simulink model "motor_ctrl_reminder"  (R2020b)
settings: Solver=VariableStepAuto  StartTime=0.0  StopTime=1  RelTol=1e-3
InitFcn:
  | Rs=0.43;
  | %Ls=31.691*1e-3;
  | Lls=0.002
  | %Rr=91.9*1e-3;
  | Rr=0.816;
  | %Lr=31.093*1e-3;
  | Llr=0.002
  | %Lm=29.897*1e-3;
  | Lm=0.6931;
  | 
  | Ls = 1.5*Lm+Lls
  | Lr = 1.5*Lm+Llr
  | 
  | Tr = Lr/Rr;
  | sigma = (Ls*Lr-Lm*Lm)/Ls/Lr;
  | 
  | J=0.085;
  | np=2;
  | 
  | Ts=1e-5;
model workspace (MAT data in the model file):
  Tsys = 2e-06
  sample_time = 1e-06
libraries: powerlib x7, simulink x2
settings Model: OrderedModelArguments=off  Creator=messer  LastModifiedBy=messer

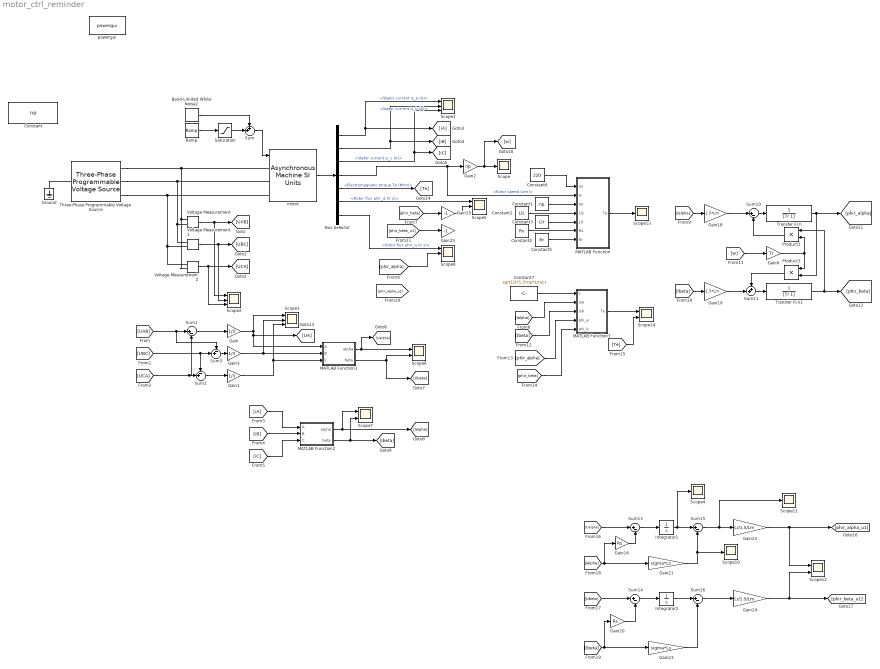
== system motor_ctrl_reminder ==
  Band-Limited White Noise2 : simulink/Sources/Band-Limited White Noise  Cov=[0.0001]  Ts=1e-4  seed=[130341]
  Bus Selector : BusSelector  OutputSignals=Stator measurements.Stator current is_a (A),Stator measurements.Stator current is_b (A),Stator measurements.Stator current is_c (A),Mechanical.Rotor speed (wm),Mechanical.Electromagnetic torque Te (N*m),Rotor measurements.Rotor flux phir_d (V s),Rotor measurements.Rotor flux phir_q (V s)
  Constant : Constant  Value=np
  Constant1 : Constant  Value=np
  Constant2 : Constant  Value=Lls
  Constant3 : Constant  Value=Llr
  Constant4 : Constant  Value=Rs
  Constant5 : Constant  Value=Rr
  Constant6 : Constant  Value=220
  Constant7 : Constant  Value=sqrt(2)*1.5*np*Lm/Lr
  Gain : Gain  Gain=1/3
  Gain1 : Gain  Gain=1/3
  Gain15 : Gain  Gain=-1
  Gain16 : Gain  Gain=Rs
  Gain18 : Gain  Gain=1.5*Lm
  Gain19 : Gain  Gain=1.5*Lm
  Gain2 : Gain  Gain=np
  Gain20 : Gain  Gain=Rs
  Gain21 : Gain  Gain=sigma*Ls
  Gain22 : Gain  Gain=Lr/1.5/Lm
  Gain23 : Gain  Gain=sigma*Ls
  Gain24 : Gain  Gain=Lr/1.5/Lm
  Gain25 : Gain  Gain=-1
  Gain3 : Gain  Gain=1/3
  Gain6 : Gain  Gain=Tr
  Ground : powerlib/Elements/Ground  LConnTagsString=a
  Integrator1 : Integrator
  Integrator2 : Integrator
  MATLAB Function : MATLAB Function  TreatAsAtomicUnit=on
  MATLAB Function1 : MATLAB Function  TreatAsAtomicUnit=on
  MATLAB Function2 : MATLAB Function  TreatAsAtomicUnit=on
  MATLAB Function3 : MATLAB Function  TreatAsAtomicUnit=on
  Product2 : Product
  Product3 : Product
  Ramp : simulink/Sources/Ramp  slope=100  start=0.25  InitialOutput=5
  Saturation : Saturate  UpperLimit=20  LowerLimit=0
  Scope{,4,10..11,13} (5 alike) : Scope
  Scope{1..3,5,8} (5 alike) : Scope  NumInputPorts=3
  Scope{6..7,12,14} (4 alike) : Scope  NumInputPorts=2
  Sum : Sum  Inputs=++|
  Sum{1,10,13..16} (6 alike) : Sum  Inputs=|+-
  Sum11 : Sum  Inputs=++|
  Sum2 : Sum  Inputs=-+|
  Sum3 : Sum  Inputs=-+|
  Three-Phase Programmable Voltage Source : powerlib/Electrical Sources/Three-Phase Programmable Voltage Source  PositiveSequence="[380/sqrt(2)  0 50]"  VariationEntity=None  VariationType=Table of time-amplitude pairs  VariationTypeAlt=Step  VariationStep=0.5  VariationRate=10  VariationMagnitude=0.3  VariationFrequency=2  VariationTiming=[1 2]  VariationPhaseA=off  Amplitudes=[1 0.8 1.2 1.0]  TimeValues=[0 0.1 0.15 0.2]  HarmonicGeneration=off  HarmonicA=[3 0.2 -25 0]  HarmonicB=[2 0.15 35 2]  Timing="[0.05  3]"  BusType=swing  Pref=0  Qref=0  Qmin=-inf  Qmax=inf
  Transfer Fcn : TransferFcn  Denominator=[Tr 1]
  Transfer Fcn1 : TransferFcn  Denominator=[Tr 1]
  Voltage Measurement : powerlib/Measurements/Voltage Measurement  PhasorSimulation=off  OutputType=Complex  PSBequivalent=0
  Voltage Measurement1 : powerlib/Measurements/Voltage Measurement  PhasorSimulation=off  OutputType=Complex  PSBequivalent=0
  Voltage Measurement2 : powerlib/Measurements/Voltage Measurement  PhasorSimulation=off  OutputType=Complex  PSBequivalent=0
  motor : powerlib/Machines/Asynchronous Machine SI Units  RotorType=Squirrel-cage  PresetModel=No  MechanicalLoad=Torque Tm  ShowDetailedParameters=on  ReferenceFrame=Stationary  Units=SI  MeasurementBus=off  NominalParameters=[1500 380 50]  Stator=[Rs Lls]  Rotor=[Rr Llr]  Cage1=[0.4155 0.002066]  Cage2=[0.4168 0.0003495]  Lm=Lm  Mechanical=[J 0 np]  PolePairs=2  InitialConditions=[1 0 0 0 0 0 0 0]  SimulateSaturation=off  Saturation=[14.03593122, 27.81365428, 53.79336849, 72.68890987, 97.98006896, 148.6815601, 215.7428561, 302.9841135, 428.7778367 ; 230, 322, 414, 460, 506, 552, 598, 644, 690]  LoadFlowParameters=1492000  TsPowergui=0  TsBlock=-1  IterativeModel=Trapezoidal non iterative  IterativeDiscreteModel=Trapezoidal non iterative  Pmec=1.492e+006
  powergui : powerlib/powergui  Priority=1  SimulationMode=Continuous  SampleTime=Tsys  frequency=60  Iterations=50  frequencyindice=50  Pbase=100e6  ErrMax=1e-4  UnitsV=kV  UnitsW=MW  buscounter=0  FunctionMessages=off  echomessages=off  EnableUseOfTLC=off  CurrentSourceSwitches=off  DisableSnubberDevices=off  DisableRonSwitches=off  DisableVfSwitches=off  DisplayEquations=off  AutomaticDiscreteSolvers=off  SolverType=Tustin/Backward Euler (TBE)  Interpol=off  ExternalGateDelay=off  methode=off  Ts=100  x0status=blocks  SPID=on  SwTol=0  HookPort=off  NonlinearTolerance=1e-4  nMaxIteration=100  ContinueOnMaxIteration=off  RestoreLinks=warning  ResistiveCurrentMeasurement=off  Frange=[0:2:500]  Ylog=off  Xlog=on  ShowGrid=off  save=off  variable=ZData  structure=0  ZoomFFT=off  StartTime=0.0  cycles=1  DisplayStyle=1  fundamental=60  FreqAxis=off  MaxFrequency=1000  frequencyindicesteady=1  RmsSteady=1  display=off
  wires:
  Bus Selector/4 -> MATLAB Function/2(w), Gain2/1  "<Rotor speed (wm)>"
  Band-Limited White Noise2/1 -> Sum/1
  Bus Selector/2 -> Scope1/2, [iB]  "<Stator current is_b (A)>"
  Bus Selector/5 -> [Te]  "<Electromagnetic torque Te (N*m)>"
  Saturation/1 -> Sum/2
  Bus Selector/1 -> [iA], Scope1/1  "<Stator current is_a (A)>"
  motor/1 -> Bus Selector/1
  Bus Selector/3 -> [iC], Scope1/3  "<Stator current is_c (A)>"
  Ramp/1 -> Saturation/1
  Voltage Measurement1/1 -> [UBC], Scope2/2
  Voltage Measurement/1 -> Scope2/1, [UAB]
  Voltage Measurement2/1 -> [UCA], Scope2/3
  [UAB] -> Sum3/1, Sum1/1
  [UCA] -> Sum1/2, Sum2/2
  Sum1/1 -> Gain/1
  [UBC] -> Sum2/1, Sum3/2
  Sum2/1 -> Gain1/1
  Sum3/1 -> Gain3/1
  Gain3/1 -> MATLAB Function1/2(B), Scope3/2
  Gain/1 -> [UA], MATLAB Function1/1(A), Scope3/1
  Gain1/1 -> MATLAB Function1/3(C), Scope3/3
  Sum/1 -> motor/1
  MATLAB Function1/1(alpha) -> [Ualpha], Scope6/1
  MATLAB Function1/2(beta) -> [Ubeta], Scope6/2
  MATLAB Function2/2(beta) -> [Ibeta], Scope7/2
  [iB] -> MATLAB Function2/2(B)
  MATLAB Function2/1(alpha) -> Scope7/1, [Ialpha]
  [Ialpha] -> Gain18/1
  Gain18/1 -> Sum10/1
  Sum10/1 -> Transfer Fcn/1
  Transfer Fcn/1 -> Product3/2, [phir_alpha]
  [Ibeta] -> Gain19/1
  Sum11/1 -> Transfer Fcn1/1
  Transfer Fcn1/1 -> Product2/1, [phir_beta]
  [w] -> Gain6/1
  Product2/1 -> Sum10/2
  Product3/1 -> Sum11/1
  Gain6/1 -> Product3/1, Product2/2
  [phir_alpha] -> Scope8/2
  [phir_beta] -> Gain15/1
  Gain15/1 -> Scope5/2
  Bus Selector/6 -> Scope5/1  "<Rotor flux phir_d (V s)>"
  Bus Selector/7 -> Scope8/1  "<Rotor flux phir_q (V s)>"
  Gain2/1 -> [w], Scope/1
  Gain19/1 -> Sum11/2
  [Ualpha] -> Sum13/1
  [Ialpha] -> Gain21/1, Gain16/1
  Gain16/1 -> Sum13/2
  [Ubeta] -> Sum14/1
  [Ibeta] -> Gain23/1, Gain20/1
  Gain20/1 -> Sum14/2
  Sum13/1 -> Integrator1/1
  Integrator1/1 -> Scope4/1, Sum15/1
  Gain21/1 -> Scope10/1, Sum15/2
  Sum15/1 -> Scope11/1, Gain22/1
  Sum14/1 -> Integrator2/1
  Integrator2/1 -> Sum16/1
  Gain23/1 -> Sum16/2
  Sum16/1 -> Gain24/1
  Gain22/1 -> [phir_alpha_u1], Scope12/1
  Gain24/1 -> [phir_beta_u1], Scope12/2
  [phir_beta_u1] -> Gain25/1
  Constant1/1 -> MATLAB Function/3(np)
  Constant2/1 -> MATLAB Function/4(Lls)
  Constant3/1 -> MATLAB Function/5(Llr)
  Constant4/1 -> MATLAB Function/6(Rs)
  Constant5/1 -> MATLAB Function/7(Rr)
  MATLAB Function/1(Te) -> Scope13/1
  Constant6/1 -> MATLAB Function/1(Us)
  [iA] -> MATLAB Function2/1(A)
  [iC] -> MATLAB Function2/3(C)
  Constant7/1 -> MATLAB Function3/1(c)
  [Ialpha] -> MATLAB Function3/2(isa)
  [Ibeta] -> MATLAB Function3/3(isb)
  [phir_alpha] -> MATLAB Function3/4(phi_a)
  [phir_beta] -> MATLAB Function3/5(phi_b)
  MATLAB Function3/1(Te) -> Scope14/1
  [Te] -> Scope14/2
  connections:
  Voltage Measurement1/LConn1 -- Voltage Measurement/LConn2 -- Three-Phase Programmable Voltage Source/RConn2 -- motor/LConn2
  Voltage Measurement2/LConn1 -- Three-Phase Programmable Voltage Source/RConn3 -- motor/LConn3 -- Voltage Measurement1/LConn2
  Voltage Measurement/LConn1 -- Voltage Measurement2/LConn2 -- Three-Phase Programmable Voltage Source/RConn1 -- motor/LConn1
  Ground/LConn1 -- Three-Phase Programmable Voltage Source/LConn1

== matlab function motor_ctrl_reminder/MATLAB Function1 ==
  data: A input; alpha output; B input; C input; beta output
function [alpha, beta] = fcn(A, B, C)
k = 2/ 3;
alpha = k * (A - 0.5*B - 0.5*C);
beta = k * sqrt(3) / 2 * (B - C);

== matlab function motor_ctrl_reminder/MATLAB Function ==
  data: Us input; w input; Te output; np input; Lls input; Llr input; Rs input; Rr input
function Te = fcn(Us, w, np,Lls, Llr, Rs, Rr)
w1 = 2*pi*50/np;
s = (w1-w)/w1;
p1 = 3*np*Us*Us*Rr/s/w1;

p2 = (Rs + Rr/s)*(Rs + Rr/s) + w1*w1*(Lls+Llr)*(Lls+Llr);

Te = p1/p2;

== matlab function motor_ctrl_reminder/MATLAB Function2 ==
  data: A input; alpha output; B input; C input; beta output
function [alpha, beta] = fcn(A, B, C)
k = 2/ 3;
alpha = k * (A - 0.5*B - 0.5*C);
beta = k * sqrt(3) / 2 * (B - C);

== matlab function motor_ctrl_reminder/MATLAB Function3 ==
  data: c input; Te output; isa input; isb input; phi_a input; phi_b input
function Te = fcn(c, isa, isb, phi_a, phi_b)
Te = c *( isb * phi_a - isa * phi_b);
